simulink model "modeloresorte"  (R2017a)
settings: Solver=VariableStepAuto  StartTime=0.0  StopTime=100  RelTol=1e-3
undefined symbols (not defined in the file or in its folder): k1, k2, k3, m1, m2
settings Model: Creator=joses  LastModifiedBy=joses

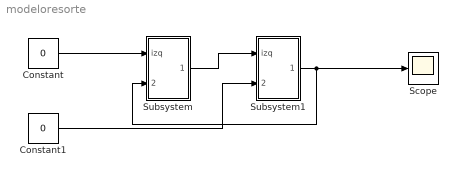
== system modeloresorte ==
  Constant : Constant  Value=0
  Constant1 : Constant  Value=0
  Scope : Scope
  Subsystem : Subsystem
  Subsystem1 : Subsystem
  wires:
  Subsystem1/1(dist) -> Scope/1, Subsystem/2(der)
  Subsystem/1(dist) -> Subsystem1/1(izq)
  Constant/1 -> Subsystem/1(izq)
  Constant1/1 -> Subsystem1/2(der)

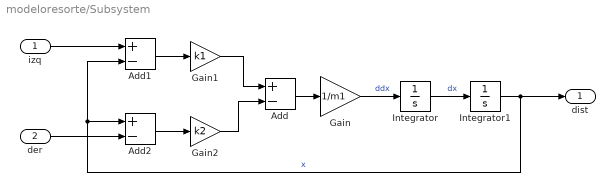
== system modeloresorte/Subsystem ==
  izq : Inport
  der : Inport  Port=2
  Add : Sum  Inputs=+-
  Add1 : Sum  Inputs=+-
  Add2 : Sum  Inputs=+-
  Gain : Gain  Gain=1/m1
  Gain1 : Gain  Gain=k1
  Gain2 : Gain  Gain=k2
  Integrator : Integrator
  Integrator1 : Integrator  InitialCondition=1
  dist : Outport
  wires:
  Add2/1 -> Gain2/1
  Gain1/1 -> Add/1
  der/1 -> Add2/2
  izq/1 -> Add1/1
  Gain/1 -> Integrator/1  "ddx"
  Integrator1/1 -> dist/1, Add2/1, Add1/2  "x"
  Integrator/1 -> Integrator1/1  "dx"
  Add1/1 -> Gain1/1
  Add/1 -> Gain/1
  Gain2/1 -> Add/2

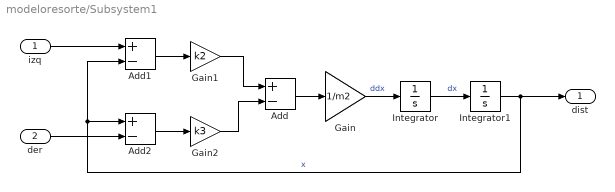
== system modeloresorte/Subsystem1 ==
  izq : Inport
  der : Inport  Port=2
  Add : Sum  Inputs=+-
  Add1 : Sum  Inputs=+-
  Add2 : Sum  Inputs=+-
  Gain : Gain  Gain=1/m2
  Gain1 : Gain  Gain=k2
  Gain2 : Gain  Gain=k3
  Integrator : Integrator
  Integrator1 : Integrator
  dist : Outport
  wires:
  Add2/1 -> Gain2/1
  Gain1/1 -> Add/1
  der/1 -> Add2/2
  izq/1 -> Add1/1
  Gain/1 -> Integrator/1  "ddx"
  Integrator1/1 -> dist/1, Add2/1, Add1/2  "x"
  Integrator/1 -> Integrator1/1  "dx"
  Add1/1 -> Gain1/1
  Add/1 -> Gain/1
  Gain2/1 -> Add/2
